simulink model "freqeuncy_v2"  (R2018b)
settings: Solver=FixedStepDiscrete  StartTime=0.0  StopTime=200e-3  FixedStep=5e-5  RelTol=1e-3
libraries: simulink x2
settings Model: Creator=enes_  LastModifiedBy=enes_
settings DataIOCC: ReturnWorkspaceOutputs=on
settings DebuggingCC: SFMachineParentedDataDiag=error

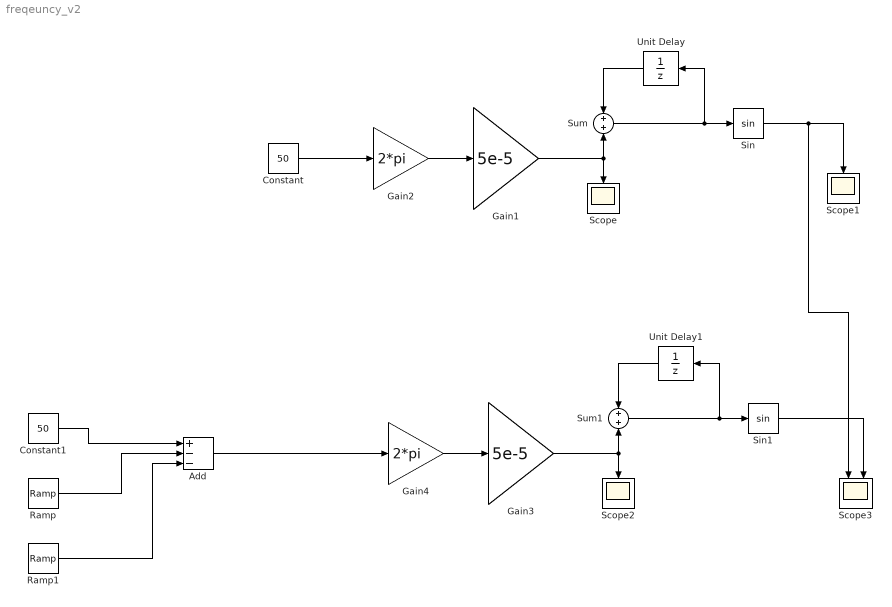
== system freqeuncy_v2 ==
  Add : Sum  Inputs=+--
  Constant : Constant  Value=50
  Constant1 : Constant  Value=50
  Gain1 : Gain  Gain=5e-5
  Gain2 : Gain  Gain=2*pi
  Gain3 : Gain  Gain=5e-5
  Gain4 : Gain  Gain=2*pi
  Ramp : simulink/Sources/Ramp  slope=0.5/100e-3  start=0  InitialOutput=0
  Ramp1 : simulink/Sources/Ramp  slope=-0.5/100e-3  start=100e-3  InitialOutput=0
  Scope : Scope
  Scope1 : Scope
  Scope2 : Scope
  Scope3 : Scope  NumInputPorts=2
  Sin : Trigonometry
  Sin1 : Trigonometry
  Sum : Sum
  Sum1 : Sum
  Unit Delay : UnitDelay  SampleTime=-1  HasFrameUpgradeWarning=on
  Unit Delay1 : UnitDelay  SampleTime=-1  HasFrameUpgradeWarning=on
  wires:
  Sum/1 -> Sin/1, Unit Delay/1
  Unit Delay/1 -> Sum/1
  Gain1/1 -> Sum/2, Scope/1
  Gain2/1 -> Gain1/1
  Sin/1 -> Scope3/1, Scope1/1
  Constant/1 -> Gain2/1
  Sin1/1 -> Scope3/2
  Unit Delay1/1 -> Sum1/1
  Sum1/1 -> Sin1/1, Unit Delay1/1
  Add/1 -> Gain4/1
  Gain3/1 -> Sum1/2, Scope2/1
  Gain4/1 -> Gain3/1
  Constant1/1 -> Add/1
  Ramp/1 -> Add/2
  Ramp1/1 -> Add/3
